simulink model "lab09_DC_Motor"  (R2022b)
settings: Solver=FixedStepAuto  StartTime=0.0  StopTime=inf  RelTol=1e-3
libraries: arduinolib x6, simulink x3
settings Model: ExtModeTrigDuration=2  Creator=MAAM  LastModifiedBy=MAAM
settings OptimizationCC: EnhancedBackFolding=on  PassReuseOutputArgsAs=Individual arguments  ZeroExternalMemoryAtStartup=off  ZeroInternalMemoryAtStartup=off  MaxStackSize=64  OptimizeBlockOrder=speed  DifferentSizesBufferReuse=on  OptimizationCustomize=off  EfficientTunableParamExpr=on
settings DebuggingCC: ParameterTunabilityLossMsg=error
settings HardwareCC: ProdBitPerInt=16  ProdBitPerPointer=16  ProdBitPerSizeT=16  ProdBitPerPtrDiffT=16  ProdLargestAtomicFloat=None  ProdWordSize=8  ProdHWDeviceType=Atmel->AVR
settings SFSimCC: MATLABDynamicMemAlloc=off
settings RTWCC: Description=Embedded Coder  SystemTargetFile=ert.tlc  HardwareBoard=Arduino Mega 2560  TemplateMakefile=ert_default_tmf  Toolchain=Arduino AVR  BuildConfiguration=Faster Runs
settings CodeAppCC: ForceParamTrailComments=on  IgnoreCustomStorageClasses=off  OperatorAnnotations=on  SimulinkDataObjDesc=on  SFDataObjDesc=on  InsertBlockDesc=on
settings ERTTargetCC: SupportContinuousTime=on  SupportVariableSizeSignals=on  ExtMode=on  ExtModeTransport=3  ExtModeStaticAlloc=on  ExtModeAutomaticAllocSize=off  ExtModeStaticAllocSize=2048  ExtModeMexFile=ext_xcp  ExtModeMexArgs=0 5 921600  ExtModeIntrfLevel=Level2 - Open

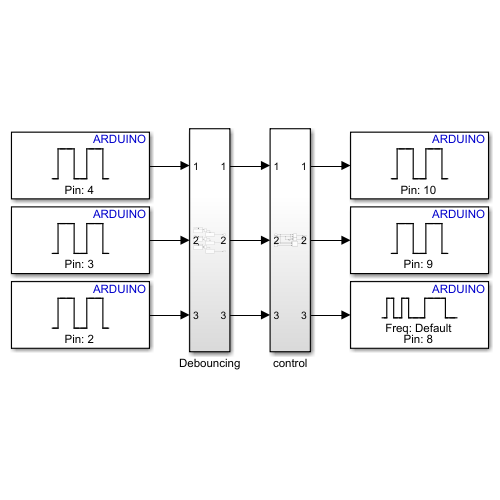
[thumbnail: Simulink's stored preview of the top-level diagram]
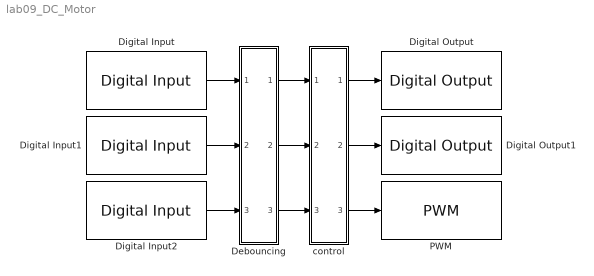
== system lab09_DC_Motor ==
  Debouncing : Subsystem
  Digital Input : arduinolib/Digital Input  pinNumber=4  mode=Default  Direction=input  SampleTime=0.1  blockPlatform=arduino
  Digital Input1 : arduinolib/Digital Input  pinNumber=3  mode=Default  Direction=input  SampleTime=0.1  blockPlatform=arduino
  Digital Input2 : arduinolib/Digital Input  pinNumber=2  mode=Default  Direction=input  SampleTime=0.1  blockPlatform=arduino
  Digital Output : arduinolib/Digital Output  pinNumber=10  Direction=output  blockPlatform=arduino
  Digital Output1 : arduinolib/Digital Output  pinNumber=9  Direction=output  blockPlatform=arduino
  PWM : arduinolib/PWM  pinNumber=8  frequencyType=Default  desiredFrequency=490.2  achievableFrequency=490.2
  control : Subsystem
  wires:
  control/2(Out2) -> Digital Output1/1
  control/1(Out1) -> Digital Output/1
  Debouncing/1(Out1) -> control/1(In1)
  Debouncing/2(Out2) -> control/2(In2)
  Debouncing/3(Out3) -> control/3(In3)
  control/3(Out3) -> PWM/1
  Digital Input/1 -> Debouncing/1(In1)
  Digital Input1/1 -> Debouncing/2(In2)
  Digital Input2/1 -> Debouncing/3(In3)

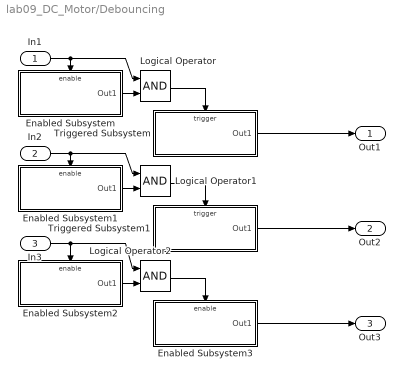
== system lab09_DC_Motor/Debouncing ==
  In1 : Inport
  In2 : Inport  Port=2
  In3 : Inport  Port=3
  Enabled Subsystem : Subsystem  TreatAsAtomicUnit=on
  Enabled Subsystem1 : Subsystem  TreatAsAtomicUnit=on
  Enabled Subsystem2 : Subsystem  TreatAsAtomicUnit=on
  Enabled Subsystem3 : Subsystem  TreatAsAtomicUnit=on
  Logical Operator : Logic  AllPortsSameDT=off  OutDataTypeStr=boolean
  Logical Operator1 : Logic  AllPortsSameDT=off  OutDataTypeStr=boolean
  Logical Operator2 : Logic  AllPortsSameDT=off  OutDataTypeStr=boolean
  Triggered Subsystem : Subsystem  TreatAsAtomicUnit=on
  Triggered Subsystem1 : Subsystem  TreatAsAtomicUnit=on
  Out1 : Outport
  Out2 : Outport  Port=2
  Out3 : Outport  Port=3
  wires:
  In1/1 -> Logical Operator/1, Enabled Subsystem/Enable
  In2/1 -> Logical Operator1/1, Enabled Subsystem1/Enable
  Enabled Subsystem/1(Out1) -> Logical Operator/2
  Enabled Subsystem1/1(Out1) -> Logical Operator1/2
  Triggered Subsystem/1(Out1) -> Out1/1
  Triggered Subsystem1/1(Out1) -> Out2/1
  In3/1 -> Logical Operator2/1, Enabled Subsystem2/Enable
  Enabled Subsystem2/1(Out1) -> Logical Operator2/2
  Enabled Subsystem3/1(Out1) -> Out3/1
  Logical Operator/1 -> Triggered Subsystem/Trigger
  Logical Operator1/1 -> Triggered Subsystem1/Trigger
  Logical Operator2/1 -> Enabled Subsystem3/Enable

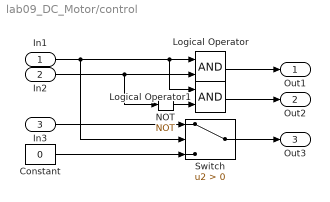
== system lab09_DC_Motor/control ==
  In1 : Inport
  In2 : Inport  Port=2
  In3 : Inport  Port=3
  Constant : Constant  Value=0
  Logical Operator : Logic  AllPortsSameDT=off  OutDataTypeStr=boolean
  Logical Operator1 : Logic  AllPortsSameDT=off  OutDataTypeStr=boolean
  NOT : Logic  Operator=NOT  IconShape=distinctive  AllPortsSameDT=off  OutDataTypeStr=boolean
  Switch : Switch  Criteria=u2 > Threshold  SaturateOnIntegerOverflow=off  InputSameDT=off
  Out1 : Outport
  Out2 : Outport  Port=2
  Out3 : Outport  Port=3
  wires:
  Constant/1 -> Switch/3
  In3/1 -> Switch/1
  In1/1 -> Logical Operator1/1, Logical Operator/1, Switch/2
  Switch/1 -> Out3/1
  Logical Operator/1 -> Out1/1
  In2/1 -> NOT/1, Logical Operator/2
  NOT/1 -> Logical Operator1/2
  Logical Operator1/1 -> Out2/1

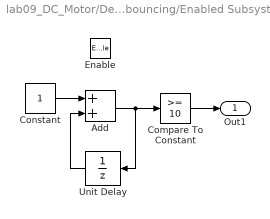
== system lab09_DC_Motor/Debouncing/Enabled Subsystem ==
  Enable : EnablePort  StatesWhenEnabling=reset
  Add : Sum
  Compare To Constant : simulink/Logic and Bit Operations/Compare To Constant  relop=>=  const=10  OutDataTypeStr=boolean
  Constant : Constant
  Unit Delay : UnitDelay  SampleTime=0.1  HasFrameUpgradeWarning=on
  Out1 : Outport
  wires:
  Constant/1 -> Add/1
  Add/1 -> Unit Delay/1, Compare To Constant/1
  Unit Delay/1 -> Add/2
  Compare To Constant/1 -> Out1/1

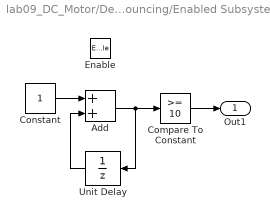
== system lab09_DC_Motor/Debouncing/Enabled Subsystem1 ==
  Enable : EnablePort  StatesWhenEnabling=reset
  Add : Sum
  Compare To Constant : simulink/Logic and Bit Operations/Compare To Constant  relop=>=  const=10  OutDataTypeStr=boolean
  Constant : Constant
  Unit Delay : UnitDelay  SampleTime=0.1  HasFrameUpgradeWarning=on
  Out1 : Outport
  wires:
  Compare To Constant/1 -> Out1/1
  Unit Delay/1 -> Add/2
  Add/1 -> Compare To Constant/1, Unit Delay/1
  Constant/1 -> Add/1

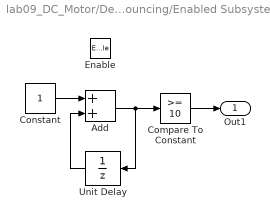
== system lab09_DC_Motor/Debouncing/Enabled Subsystem2 ==
  Enable : EnablePort  StatesWhenEnabling=reset
  Add : Sum
  Compare To Constant : simulink/Logic and Bit Operations/Compare To Constant  relop=>=  const=10  OutDataTypeStr=boolean
  Constant : Constant
  Unit Delay : UnitDelay  SampleTime=0.1  HasFrameUpgradeWarning=on
  Out1 : Outport
  wires:
  Constant/1 -> Add/1
  Add/1 -> Unit Delay/1, Compare To Constant/1
  Unit Delay/1 -> Add/2
  Compare To Constant/1 -> Out1/1

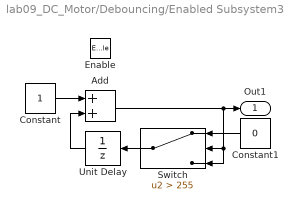
== system lab09_DC_Motor/Debouncing/Enabled Subsystem3 ==
  Enable : EnablePort
  Add : Sum
  Constant : Constant
  Constant1 : Constant  Value=0
  Switch : Switch  Criteria=u2 > Threshold  Threshold=255  SaturateOnIntegerOverflow=off  InputSameDT=off
  Unit Delay : UnitDelay  HasFrameUpgradeWarning=on
  Out1 : Outport
  wires:
  Add/1 -> Switch/2, Switch/3, Out1/1
  Unit Delay/1 -> Add/2
  Constant/1 -> Add/1
  Switch/1 -> Unit Delay/1
  Constant1/1 -> Switch/1

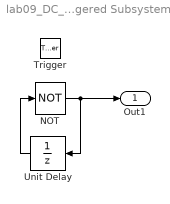
== system lab09_DC_Motor/Debouncing/Triggered Subsystem ==
  Trigger : TriggerPort  VariantControl=(inherit)
  NOT : Logic  Operator=NOT  IconShape=distinctive  AllPortsSameDT=off  OutDataTypeStr=boolean
  Unit Delay : UnitDelay  SampleTime=-1  HasFrameUpgradeWarning=on
  Out1 : Outport
  wires:
  Unit Delay/1 -> NOT/1
  NOT/1 -> Unit Delay/1, Out1/1

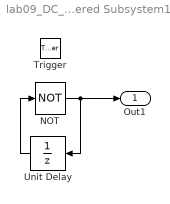
== system lab09_DC_Motor/Debouncing/Triggered Subsystem1 ==
  Trigger : TriggerPort  VariantControl=(inherit)
  NOT : Logic  Operator=NOT  IconShape=distinctive  AllPortsSameDT=off  OutDataTypeStr=boolean
  Unit Delay : UnitDelay  SampleTime=-1  HasFrameUpgradeWarning=on
  Out1 : Outport
  wires:
  NOT/1 -> Out1/1, Unit Delay/1
  Unit Delay/1 -> NOT/1
